simulink model "hosmc_sim"  (Simulink 9.2)
settings: Solver=ode4  StartTime=0.0  StopTime=5  FixedStep=0.001  RelTol=1e-3
settings Model: Creator=rosfun  LastModifiedBy=rosfun  ExtModeTrigMode=oneshot  ExtModeArmWhenConnect=off
settings DataIOCC: LimitDataPoints=off
settings OptimizationCC: BlockReduction=off  BooleanDataType=off  LifeSpan=auto
settings DebuggingCC: SaveWithParameterizedLinksMsg=none  SignalResolutionControl=TryResolveAllWithWarning  MultiTaskDSMMsg=warning  MultiTaskCondExecSysMsg=none  FcnCallInpInsideContextMsg=error  StateNameClashWarn=none  SFUnexpectedBacktrackingDiag=error  SFNoUnconditionalDefaultTransitionDiag=error  SFExecutionAtInitializationDiag=warning
settings HardwareCC: ProdBitPerPointer=64  ProdBitPerSizeT=64  ProdBitPerPtrDiffT=64  ProdLargestAtomicFloat=Float  ProdIntDivRoundTo=Zero  ProdEndianess=LittleEndian  ProdWordSize=64  ProdHWDeviceType=Intel->x86-64 (Windows64)  TargetUnknown=on
settings SFSimCC: SimUseLocalCustomCode=on
settings RTWCC: RTWUseLocalCustomCode=on
settings CodeAppCC: StateflowObjectComments=off
settings GRTTargetCC: TargetLangStandard=C99 (ISO)  GeneratePreprocessorConditionals=Use local settings
settings ConfigComp: CovMetricSettings=dwe  CovHtmlReporting=off  CovSaveCumulativeToWorkspaceVar=off  CovSaveSingleToWorkspaceVar=off  CovExternalEMLEnable=on

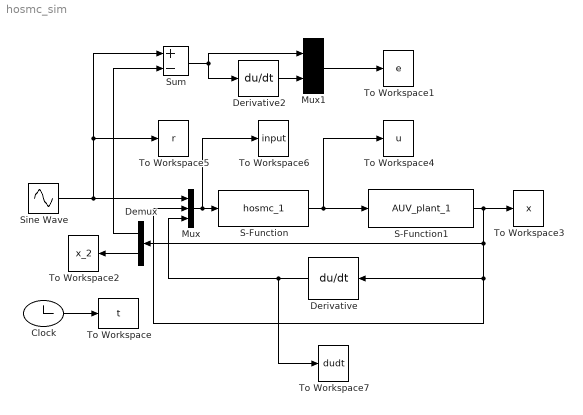
== system hosmc_sim ==
  Clock : Clock
  Demux : Demux  Outputs=2
  Derivative : Derivative
  Derivative2 : Derivative
  Mux : Mux  Inputs=3
  Mux1 : Mux  Inputs=2
  S-Function : S-Function  FunctionName=hosmc_1  SFunctionDeploymentMode=off  EnableBusSupport=off
  S-Function1 : S-Function  FunctionName=AUV_plant_1  SFunctionDeploymentMode=off  EnableBusSupport=off
  Sine Wave : Sin  Amplitude=0.5  Bias=pi/6  Frequency=2*pi  SampleTime=0
  Sum : Sum  Inputs=+-  SaturateOnIntegerOverflow=on  InputSameDT=on  OutDataTypeStr=Inherit: Same as first input
  To Workspace : ToWorkspace  VariableName=t  SampleTime=-1
  To Workspace1 : ToWorkspace  VariableName=e  SampleTime=-1
  To Workspace2 : ToWorkspace  VariableName=x_2  SampleTime=-1
  To Workspace3 : ToWorkspace  VariableName=x  SampleTime=-1
  To Workspace4 : ToWorkspace  VariableName=u  SampleTime=-1
  To Workspace5 : ToWorkspace  VariableName=r  SampleTime=-1
  To Workspace6 : ToWorkspace  VariableName=input  SampleTime=-1
  To Workspace7 : ToWorkspace  VariableName=dudt  SampleTime=-1
  wires:
  Mux/1 -> To Workspace6/1, S-Function/1
  S-Function1/1 -> Mux/2, Derivative/1, Demux/1, To Workspace3/1
  Clock/1 -> To Workspace/1
  S-Function/1 -> S-Function1/1, To Workspace4/1
  Derivative/1 -> To Workspace7/1, Mux/3
  Sine Wave/1 -> Mux/1, Sum/1, To Workspace5/1
  Sum/1 -> Derivative2/1, Mux1/1
  Derivative2/1 -> Mux1/2
  Mux1/1 -> To Workspace1/1
  Demux/1 -> Sum/2
  Demux/2 -> To Workspace2/1
